simulink subsystem "convertRawAccel"  (R2024a)
settings: Solver=VariableStepAuto  StartTime=0.0  StopTime=10.0  RelTol=1e-3
libraries: hdlsllib x3, simulink x3
settings Model: Creator=Peter  LastModifiedBy=Peter

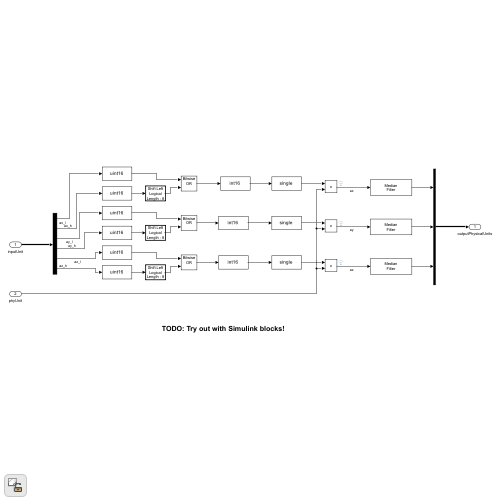
[thumbnail: Simulink's stored preview of the top-level diagram]
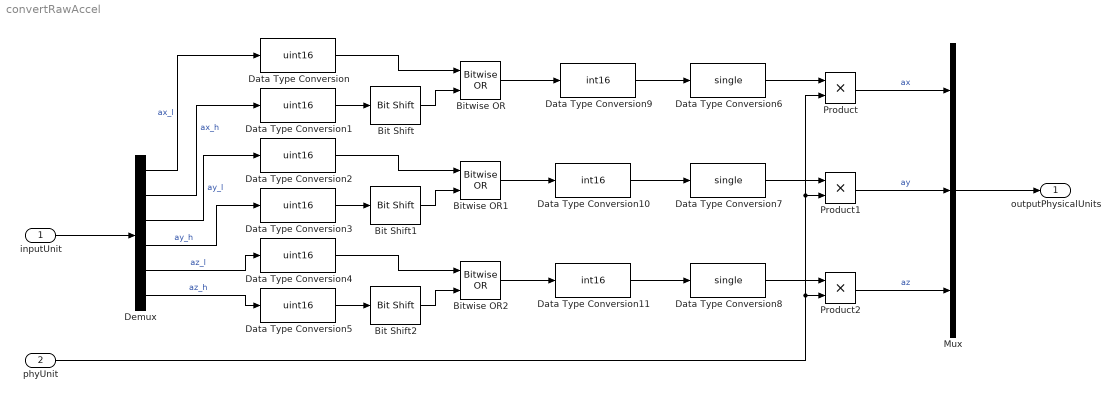
== system convertRawAccel ==
  inputUnit : Inport  OutDataTypeStr=fixdt('uint8', 'DataTypeOverride', 'Off')
  phyUnit : Inport  Port=2
  Bit Shift : hdlsllib/Logic and Bit Operations/Bit Shift  mode=Shift Left Logical  N=8
  Bit Shift1 : hdlsllib/Logic and Bit Operations/Bit Shift  mode=Shift Left Logical  N=8
  Bit Shift2 : hdlsllib/Logic and Bit Operations/Bit Shift  mode=Shift Left Logical  N=8
  Bitwise OR : simulink/Logic and Bit Operations/Bitwise Operator  logicop=OR  UseBitMask=off  NumInputPorts=2  BitMask=bin2dec('11011001')  BitMaskRealWorld=Stored Integer
      settings: LibrarySourceBlock=|
      | simulink/Quick Insert/Logic and Bit
      | Operations/Bitwise OR
  Bitwise OR1 : simulink/Logic and Bit Operations/Bitwise Operator  logicop=OR  UseBitMask=off  NumInputPorts=2  BitMask=bin2dec('11011001')  BitMaskRealWorld=Stored Integer
      settings: LibrarySourceBlock=|
      | simulink/Quick Insert/Logic and Bit
      | Operations/Bitwise OR
  Bitwise OR2 : simulink/Logic and Bit Operations/Bitwise Operator  logicop=OR  UseBitMask=off  NumInputPorts=2  BitMask=bin2dec('11011001')  BitMaskRealWorld=Stored Integer
      settings: LibrarySourceBlock=|
      | simulink/Quick Insert/Logic and Bit
      | Operations/Bitwise OR
  Data Type Conversion{,1..5} (6 alike) : DataTypeConversion  OutDataTypeStr=uint16  ConvertRealWorld=Stored Integer (SI)  SaturateOnIntegerOverflow=off  RndMeth=Floor
  Data Type Conversion10 : DataTypeConversion  OutDataTypeStr=int16  ConvertRealWorld=Stored Integer (SI)  SaturateOnIntegerOverflow=off  RndMeth=Floor
  Data Type Conversion11 : DataTypeConversion  OutDataTypeStr=int16  ConvertRealWorld=Stored Integer (SI)  SaturateOnIntegerOverflow=off  RndMeth=Floor
  Data Type Conversion6 : DataTypeConversion  OutDataTypeStr=single  SaturateOnIntegerOverflow=off  RndMeth=Floor
  Data Type Conversion7 : DataTypeConversion  OutDataTypeStr=single  SaturateOnIntegerOverflow=off  RndMeth=Floor
  Data Type Conversion8 : DataTypeConversion  OutDataTypeStr=single  SaturateOnIntegerOverflow=off  RndMeth=Floor
  Data Type Conversion9 : DataTypeConversion  OutDataTypeStr=int16  ConvertRealWorld=Stored Integer (SI)  SaturateOnIntegerOverflow=off  RndMeth=Floor
  Demux : Demux  Outputs=6
  Mux : Mux  Inputs=3
  Product : Product
  Product1 : Product
  Product2 : Product
  outputPhysicalUnits : Outport
  wires:
  Demux/5 -> Data Type Conversion4/1  "az_l"
  Demux/6 -> Data Type Conversion5/1  "az_h"
  Demux/2 -> Data Type Conversion1/1  "ax_h"
  Demux/3 -> Data Type Conversion2/1  "ay_l"
  Demux/1 -> Data Type Conversion/1  "ax_l"
  Demux/4 -> Data Type Conversion3/1  "ay_h"
  phyUnit/1 -> Product2/2, Product/2, Product1/2
  inputUnit/1 -> Demux/1
  Bit Shift/1 -> Bitwise OR/2
  Data Type Conversion/1 -> Bitwise OR/1
  Data Type Conversion1/1 -> Bit Shift/1
  Product1/1 -> Mux/2  "ay"
  Product/1 -> Mux/1  "ax"
  Product2/1 -> Mux/3  "az"
  Mux/1 -> outputPhysicalUnits/1
  Bitwise OR/1 -> Data Type Conversion9/1
  Bitwise OR1/1 -> Data Type Conversion10/1
  Data Type Conversion3/1 -> Bit Shift1/1
  Data Type Conversion2/1 -> Bitwise OR1/1
  Bit Shift1/1 -> Bitwise OR1/2
  Bit Shift2/1 -> Bitwise OR2/2
  Data Type Conversion4/1 -> Bitwise OR2/1
  Data Type Conversion5/1 -> Bit Shift2/1
  Bitwise OR2/1 -> Data Type Conversion11/1
  Data Type Conversion6/1 -> Product/1
  Data Type Conversion7/1 -> Product1/1
  Data Type Conversion8/1 -> Product2/1
  Data Type Conversion9/1 -> Data Type Conversion6/1
  Data Type Conversion10/1 -> Data Type Conversion7/1
  Data Type Conversion11/1 -> Data Type Conversion8/1
